simulink model "sampleModel288"  (R2021b)
settings: Solver=VariableStepAuto  StartTime=0.0  StopTime=10.0  RelTol=1e-3
undefined symbols (not defined in the file or in its folder): Newton, Raphson
libraries: simulink x1
settings Model: Creator=user  LastModifiedBy=user

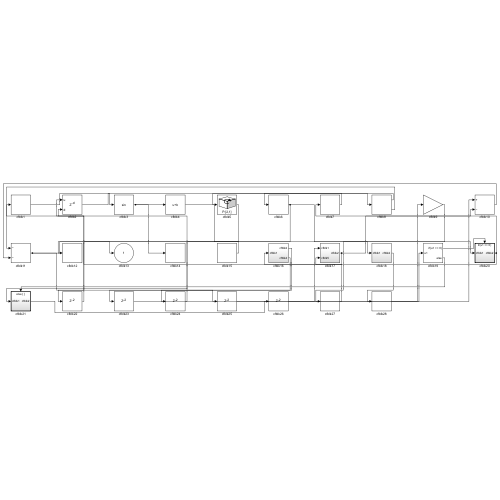
[thumbnail: Simulink's stored preview of the top-level diagram]
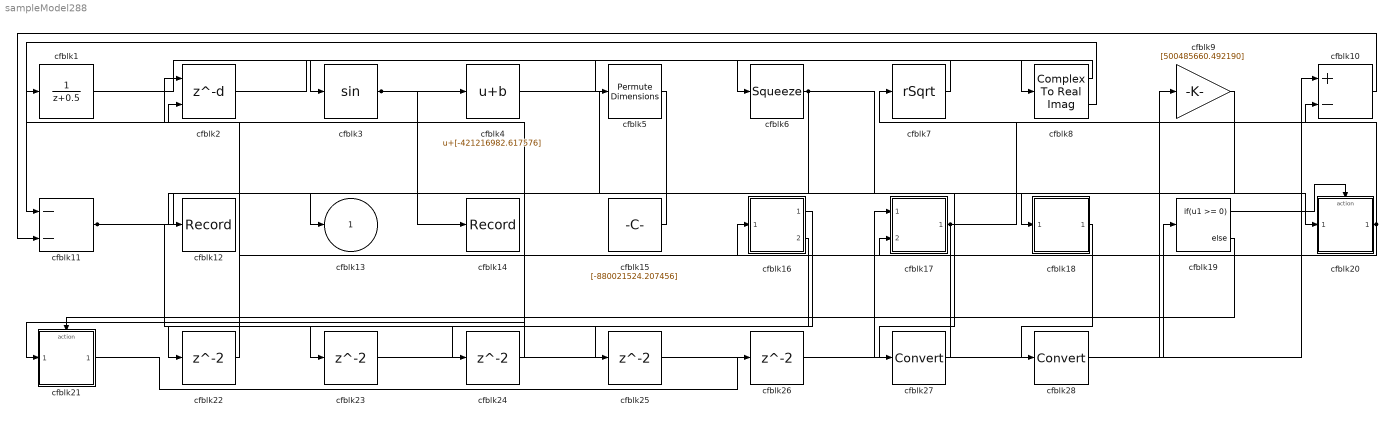
== system sampleModel288 ==
  cfblk1 : DiscreteTransferFcn  SampleTime=1
  cfblk10 : Sum  Inputs=+-
  cfblk11 : Sum  Inputs=--
  cfblk12 : Record  FileSettingsInternal="{\"entries\":[{\"content\":{\"excelSettings\":{\"content\":{},\"type\":\"Streamout.ExcelSettings\"}},\"type\":\"Streamout.FileSettingStorage\",\"uuid\":\"99121057-6bef-407f-aaef-170d9c7b3167\"}],\"packageUris\":[\"http://schema.mathworks.com/mf0/streamout_blocks/R2020a\"],\"version\":\"1.0\"}"  SignalsInternal="{\"entries\":[{\"content\":{\"signals\":[{\"content\":{\"blockPath\":[\"sampleModel288/cfblk12\"],\"channel\":[],\"dimensions\":[1],\"domain\":\"sampleModel288/cfblk12\",\"lineColor\":\"#fe330a\",\"plots\":[1],\"port\":1,\"sid\":[\"\"],\"signalID\":12254,\"signalName\":\"cfblk15\"},\"type\":\"RecordBlkView.Signal\",\"uuid\":\"5aa2cc36-c58b-4dea-8277-25bc0cf200c1\"}]},\"type\":\"RecordBlkView.InputSignals\",\"uuid\":\"3db44b6d-059e-402a-99a5-882ccea2dec7\"}],\"packageUris\":[\"http://schema.mathworks.com/mf0/streamout_blocks/R2020a\"],\"version\":\"1.0\"}"  VisualizationBindings="{\"sparklinesplugin\":{\"info\":[{\"bindingParametersList\":[],\"subplotID\":1}]}}"
  cfblk14 : Record  FileSettingsInternal="{\"entries\":[{\"content\":{\"excelSettings\":{\"content\":{},\"type\":\"Streamout.ExcelSettings\"}},\"type\":\"Streamout.FileSettingStorage\",\"uuid\":\"4ec19c18-7a8b-4270-a29a-3678415878d8\"}],\"packageUris\":[\"http://schema.mathworks.com/mf0/streamout_blocks/R2020a\"],\"version\":\"1.0\"}"  SignalsInternal="{\"entries\":[{\"content\":{\"signals\":[{\"content\":{\"blockPath\":[\"sampleModel288/cfblk14\"],\"channel\":[],\"dimensions\":[1],\"domain\":\"sampleModel288/cfblk14\",\"lineColor\":\"#ff13a6\",\"plots\":[1],\"port\":1,\"sid\":[\"\"],\"signalID\":12250,\"signalName\":\"cfblk3\"},\"type\":\"RecordBlkView.Signal\",\"uuid\":\"5c43b3db-2ae5-42b3-9552-7b278d10c03a\"}]},\"type\":\"RecordBlkView.InputSignals\",\"uuid\":\"71f823b3-9054-4343-a0f3-88d36fe46df6\"}],\"packageUris\":[\"http://schema.mathworks.com/mf0/streamout_blocks/R2020a\"],\"version\":\"1.0\"}"  VisualizationBindings="{\"sparklinesplugin\":{\"info\":[{\"bindingParametersList\":[],\"subplotID\":1}]}}"
  cfblk15 : Constant  Value=[-880021524.207456]  SampleTime=1
  cfblk16 : Subsystem
  cfblk17 : Subsystem
  cfblk18 : Subsystem
  cfblk19 : If  IfExpression=u1 >= 0  SampleTime=1
  cfblk2 : Delay  DelayLengthSource=Input port  SampleTime=1
      settings: InputPortMap=u0,p1
  cfblk20 : Subsystem  TreatAsAtomicUnit=on
  cfblk21 : Subsystem  TreatAsAtomicUnit=on
  cfblk{22..26} (5 alike) : Delay  SampleTime=1
  cfblk27 : DataTypeConversion
  cfblk28 : DataTypeConversion
  cfblk3 : Trigonometry
  cfblk4 : Bias  Bias=[-421216982.617576]
  cfblk5 : PermuteDimensions
  cfblk6 : Squeeze
  cfblk7 : Sqrt  Operator=rSqrt  AlgorithmType=Newton-Raphson  SaturateOnIntegerOverflow=on
  cfblk8 : ComplexToRealImag
  cfblk9 : Gain  Gain=[500485660.492190]
  cfblk13 : Outport
  wires:
  cfblk1/1 -> cfblk3/1
  cfblk3/1 -> cfblk14/1, cfblk4/1
  cfblk11/1 -> cfblk13/1, cfblk25/1
  cfblk6/1 -> cfblk21/1(cfblk1), cfblk20/1(cfblk1)
  cfblk8/1 -> cfblk6/1
  cfblk2/1 -> cfblk8/1
  cfblk8/2 -> cfblk11/1
  cfblk4/1 -> cfblk18/1(cfblk1)
  cfblk7/1 -> cfblk5/1
  cfblk17/1(cfblk2) -> cfblk16/1(cfblk1), cfblk10/2
  cfblk10/1 -> cfblk11/2
  cfblk15/1 -> cfblk12/1
  cfblk20/1(cfblk2) -> cfblk7/1, cfblk17/2(cfblk5)
  cfblk19/1 -> cfblk20/Action
  cfblk19/2 -> cfblk21/Action
  cfblk5/1 -> cfblk22/1
  cfblk22/1 -> cfblk2/1
  cfblk16/1(cfblk2) -> cfblk23/1
  cfblk23/1 -> cfblk17/1(cfblk1)
  cfblk16/2(cfblk4) -> cfblk24/1
  cfblk24/1 -> cfblk1/1
  cfblk25/1 -> cfblk10/1
  cfblk21/1(cfblk2) -> cfblk26/1
  cfblk26/1 -> cfblk19/1
  cfblk9/1 -> cfblk27/1
  cfblk27/1 -> cfblk2/2
  cfblk18/1(cfblk2) -> cfblk28/1
  cfblk28/1 -> cfblk9/1

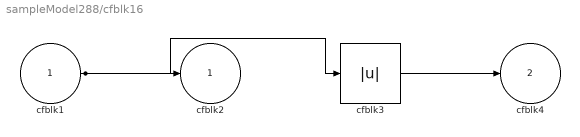
== system sampleModel288/cfblk16 ==
  cfblk1 : Inport
  cfblk3 : Abs
  cfblk2 : Outport
  cfblk4 : Outport  Port=2
  wires:
  cfblk1/1 -> cfblk3/1, cfblk2/1
  cfblk3/1 -> cfblk4/1

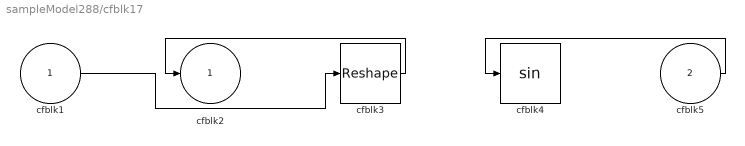
== system sampleModel288/cfblk17 ==
  cfblk1 : Inport
  cfblk5 : Inport  Port=2
  cfblk3 : Reshape
  cfblk4 : Trigonometry
  cfblk2 : Outport
  wires:
  cfblk3/1 -> cfblk2/1
  cfblk1/1 -> cfblk3/1
  cfblk5/1 -> cfblk4/1

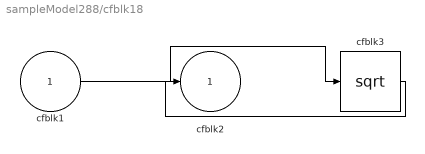
== system sampleModel288/cfblk18 ==
  cfblk1 : Inport
  cfblk3 : Sqrt  SaturateOnIntegerOverflow=on
  cfblk2 : Outport
  wires:
  cfblk1/1 -> cfblk3/1
  cfblk3/1 -> cfblk2/1

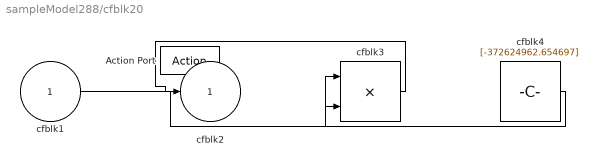
== system sampleModel288/cfblk20 ==
  cfblk1 : Inport
  Action Port : ActionPort  ActionPortLabel=if(u1 >= 0)
  cfblk3 : Product  Inputs=**
  cfblk4 : Constant  Value=[-372624962.654697]  SampleTime=1
  cfblk2 : Outport
  wires:
  cfblk1/1 -> cfblk3/1
  cfblk4/1 -> cfblk3/2
  cfblk3/1 -> cfblk2/1

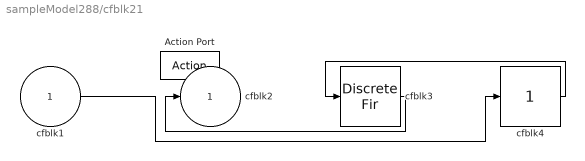
== system sampleModel288/cfblk21 ==
  cfblk1 : Inport
  Action Port : ActionPort  ActionPortLabel=else
  cfblk3 : DiscreteFir
  cfblk4 : simulink/Math Operations/Slider Gain  gain=1  low=0  high=2
  cfblk2 : Outport
  wires:
  cfblk3/1 -> cfblk2/1
  cfblk1/1 -> cfblk4/1
  cfblk4/1 -> cfblk3/1
